simulink model "ctrlStarter"  (R2022a)
settings: Solver=FixedStepAuto  StartTime=0.0  StopTime=180  FixedStep=Ts  RelTol=1e-3
undefined symbols (not defined in the file or in its folder): ctrl2TwinStruct, ctrlSignal1, ctrlSignal2, ctrlSignal3, ctrlSignal4, ctrlSignalStruct, curAft, curBow
settings Model: Creator=EGI-Z400  LastModifiedBy=jspin
settings DebuggingCC: UnconnectedInputMsg=warning  UnconnectedOutputMsg=warning  UnconnectedLineMsg=warning
settings RTWCC: Description=Generic Real-Time Target  DLArmComputeVersion=19.05

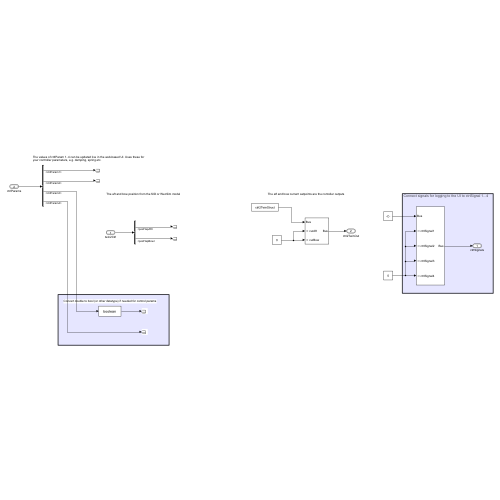
[thumbnail: Simulink's stored preview of the top-level diagram]
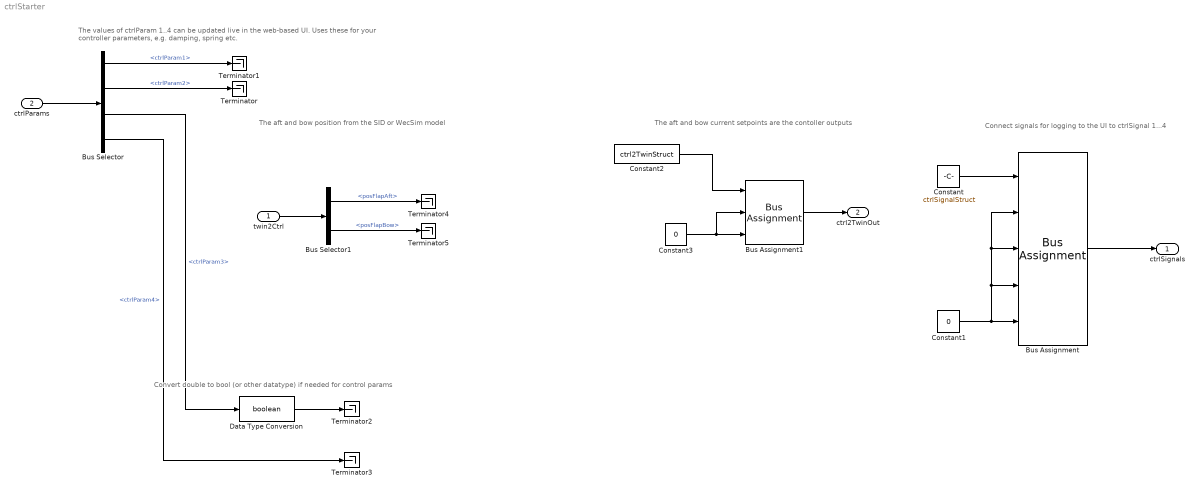
== system ctrlStarter ==
  note: The aft and bow current setpoints are the contoller outputs
  note: The values of ctrlParam 1..4 can be updated live in the web-based UI. Uses these for your controller parameters, e.g. damping, spring etc.
  note: The aft and bow position from the SID or WecSim model
  note: Convert double to bool (or other datatype) if needed for control params
  note: Connect signals for logging to the UI to ctrlSignal 1...4
  twin2Ctrl : Inport  OutDataTypeStr=Bus: twin2CtrlBus
  ctrlParams : Inport  Port=2  OutDataTypeStr=Bus: ctrlParamBus
  Bus Assignment : BusAssignment  AssignedSignals=ctrlSignal1,ctrlSignal2,ctrlSignal3,ctrlSignal4
  Bus Assignment1 : BusAssignment  AssignedSignals=curAft,curBow
  Bus Selector : BusSelector  OutputSignals=ctrlParam1,ctrlParam2,ctrlParam3,ctrlParam4
  Bus Selector1 : BusSelector  OutputSignals=posFlapAft,posFlapBow
  Constant : Constant  Value=ctrlSignalStruct  OutDataTypeStr=Bus: ctrlSignalBus
  Constant1 : Constant  Value=0
  Constant2 : Constant  Value=ctrl2TwinStruct  OutDataTypeStr=Bus: ctrl2TwinBus
  Constant3 : Constant  Value=0
  Data Type Conversion : DataTypeConversion  OutDataTypeStr=boolean  SaturateOnIntegerOverflow=off  RndMeth=Floor
  Terminator{,1..5} (6 alike) : Terminator
  ctrlSignals : Outport  OutDataTypeStr=Bus: ctrlSignalBus
  ctrl2TwinOut : Outport  Port=2  OutDataTypeStr=Bus: ctrl2TwinBus
  wires:
  Data Type Conversion/1 -> Terminator2/1
  ctrlParams/1 -> Bus Selector/1
  Bus Selector/1 -> Terminator1/1  "<ctrlParam1>"
  Bus Selector/2 -> Terminator/1  "<ctrlParam2>"
  Bus Selector/3 -> Data Type Conversion/1  "<ctrlParam3>"
  Bus Selector/4 -> Terminator3/1  "<ctrlParam4>"
  Constant/1 -> Bus Assignment/1
  Bus Assignment/1 -> ctrlSignals/1
  Constant1/1 -> Bus Assignment/2, Bus Assignment/3, Bus Assignment/4, Bus Assignment/5
  twin2Ctrl/1 -> Bus Selector1/1
  Bus Selector1/1 -> Terminator4/1  "<posFlapAft>"
  Bus Selector1/2 -> Terminator5/1  "<posFlapBow>"
  Bus Assignment1/1 -> ctrl2TwinOut/1
  Constant2/1 -> Bus Assignment1/1
  Constant3/1 -> Bus Assignment1/2, Bus Assignment1/3
